simulink subsystem "iLBCTransmit"  (R2024b)
settings: Solver=VariableStepAuto  StartTime=0.0  StopTime=10.0  RelTol=1e-3
values from neighbouring files (symbols this model uses):
  in = pn()    [waveform_generator_Preamble.m]
  LSF = hexToArray(LSF,1)    [Full_transmit.m]
undefined symbols (not defined in the file or in its folder): dspblkCoreblockFVToolHelper, gcbh, ilbc, ilbcMode
libraries: simulink x19, matrix_library x13, dspmtrx3 x9, dspquant2 x6, dspilbclib x5, dspstat3 x5, dspsigops x5, simulink_need_slupdate x2, audiosources x1, dsplp x1, dspsolvers x1
(part 2 of 2)

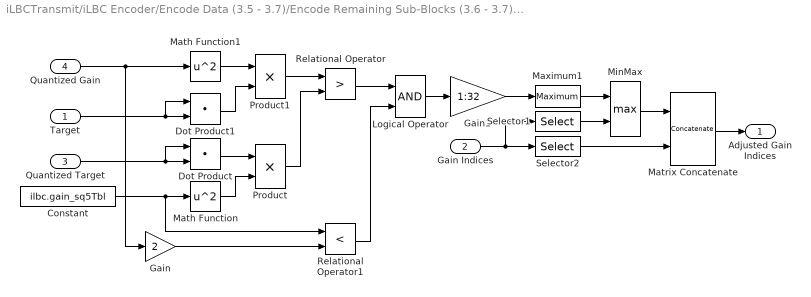
== system iLBCTransmit/iLBC Encoder/Encode Data (3.5 - 3.7)/Encode Remaining Sub-Blocks (3.6 - 3.7)/Encode Sub-Block (3.6.2 - 3.7)/Adjust First Gain Index (3.7) ==
  Target : Inport
  Gain Indices : Inport  Port=2
  Quantized Target : Inport  Port=3
  Quantized Gain : Inport  Port=4
  Constant : Constant  Value=ilbc.gain_sq5Tbl  VectorParams1D=off  OutDataTypeStr=Inherit: Inherit via back propagation
  Dot Product : DotProduct  OutDataTypeStr=Inherit: Inherit via internal rule
  Dot Product1 : DotProduct  OutDataTypeStr=Inherit: Inherit via internal rule
  Gain : Gain  Gain=2
  Gain1 : Gain  Gain=1:32  OutDataTypeStr=Inherit: Inherit via back propagation
  Logical Operator : Logic  AllPortsSameDT=off  OutDataTypeStr=uint(8)
  Math Function : Math  Operator=square  SignedPower=on
  Math Function1 : Math  Operator=square  SignedPower=on
  Matrix Concatenate : Concatenate  Mode=Multidimensional array
  Maximum1 : dspstat3/Maximum  operation=maximum  fcn=Index  indexBase=Zero  operateOver=Each row  Dimension=1  InputProcessing=Columns as channels (frame based)  reset=None  roiEnable=off  roiType=Rectangles  roiPortion=Entire ROI  roiOutput=Individual statistics for each ROI  roiFlag=off  roundingMode=Floor  overflowMode=off  accumDataTypeStr=Inherit: Same as product output  accumLastDataTypeStr=Inherit: Same as product output
  MinMax : MinMax  Function=max  Inputs=2  OutDataTypeStr=Inherit: Inherit via back propagation
  Product : Product  RndMeth=Zero
  Product1 : Product  RndMeth=Zero
  Relational Operator : RelationalOperator  Operator=>  OutDataTypeStr=uint(8)  InputSameDT=off
  Relational Operator1 : RelationalOperator  Operator=<  OutDataTypeStr=uint(8)  InputSameDT=off
  Selector1 : Selector  NumberOfDimensions=2  InputPortWidth=151  IndexOptions=Index vector (dialog),Select all  Indices=1,1  OutputSizes=1,1
  Selector2 : Selector  NumberOfDimensions=2  InputPortWidth=151  IndexOptions=Index vector (dialog),Select all  Indices=2:3,1  OutputSizes=1,1
  Adjusted Gain Indices : Outport  VectorParamsAs1DForOutWhenUnconnected=off
  wires:
  Gain1/1 -> Maximum1/1
  Logical Operator/1 -> Gain1/1
  Relational Operator1/1 -> Logical Operator/2
  Relational Operator/1 -> Logical Operator/1
  Gain/1 -> Relational Operator1/2
  Product/1 -> Relational Operator/2
  Product1/1 -> Relational Operator/1
  Target/1 -> Dot Product1/1, Dot Product1/2
  Quantized Target/1 -> Dot Product/1, Dot Product/2
  Quantized Gain/1 -> Gain/1, Math Function1/1
  Dot Product1/1 -> Product1/2
  Math Function1/1 -> Product1/1
  Dot Product/1 -> Product/1
  Math Function/1 -> Product/2
  Constant/1 -> Relational Operator1/1, Math Function/1
  Matrix Concatenate/1 -> Adjusted Gain Indices/1
  MinMax/1 -> Matrix Concatenate/1
  Maximum1/1 -> MinMax/1
  Selector1/1 -> MinMax/2
  Selector2/1 -> Matrix Concatenate/2
  Gain Indices/1 -> Selector2/1, Selector1/1

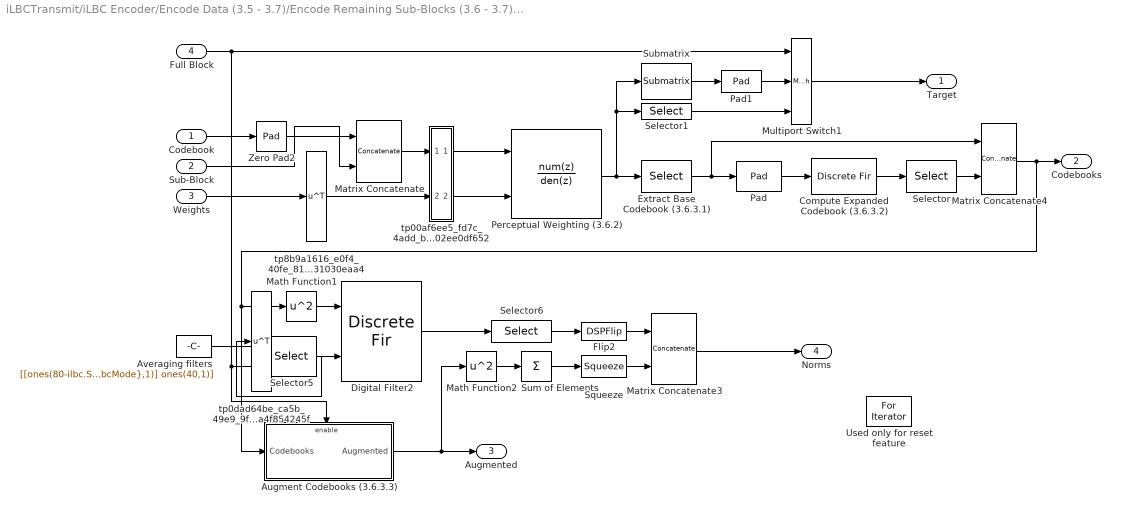
== system iLBCTransmit/iLBC Encoder/Encode Data (3.5 - 3.7)/Encode Remaining Sub-Blocks (3.6 - 3.7)/Encode Sub-Block (3.6.2 - 3.7)/Compute Codebooks (3.6.2 - 3.6.3) ==
  Codebook : Inport
  Sub-Block : Inport  Port=2
  Weights : Inport  Port=3
  Full Block : Inport  Port=4
  Augment Codebooks (3.6.3.3) : Subsystem
  Averaging filters : Constant  Value=[[ones(80-ilbc.STATE_SHORT_LEN{ilbcMode},1); zeros(40-80+ilbc.STATE_SHORT_LEN{ilbcMode},1)] ones(40,1)]  OutDataTypeStr=Inherit: Inherit via back propagation
  Compute Expanded Codebook (3.6.3.2) : DiscreteFir  Coefficients=ilbc.cbfiltersTbl  InputProcessing=Columns as channels (frame based)  AccumDataTypeStr=Inherit: Same as product output
  Digital Filter2 : DiscreteFir  CoefSource=Input port  Coefficients=[1 2]  InputProcessing=Columns as channels (frame based)  AccumDataTypeStr=Inherit: Same as product output
      settings: InputPortMap=u0,u1
  Extract Base Codebook (3.6.3.1) : Selector  NumberOfDimensions=2  InputPortWidth=151  IndexOptions=Index vector (dialog),Index vector (dialog)  Indices=1:147,1  OutputSizes=1,1
  Flip2 : DSPFlip
  Math Function1 : Math  Operator=square  SignedPower=on
  Math Function2 : Math  Operator=square  SignedPower=on
  Matrix Concatenate : Concatenate  Mode=Multidimensional array
  Matrix Concatenate3 : Concatenate  Mode=Multidimensional array
  Matrix Concatenate4 : Concatenate  Mode=Multidimensional array  ConcatenateDimension=2
  Multiport Switch1 : MultiPortSwitch  DataPortOrder=Zero-based contiguous  Inputs=2  zeroidx=on  SaturateOnIntegerOverflow=off  InputSameDT=off
  Pad : dspsigops/Pad  padAlong=Specified dimensions  dimsToPad=1  valSrc=Specify via dialog  padVal=0  spec=Pad size  padNumOutRowsSpecMethod=User-specified  numOutRows=1  padNumOutColsSpecMethod=User-specified  numOutCols=1  isVarDimsMode=off  padBeginning=0  padEnd=4  outSizeMode=User-specified  outSize=1  padSigAt=End  trunc_flag=None  roundingMode=Floor  overflowMode=off  truncOrWrapMode=Truncate  wrap_flag=None
  Pad1 : dspsigops/Pad  padAlong=Columns  dimsToPad=1  valSrc=Specify via dialog  padVal=0  spec=Output size  padNumOutRowsSpecMethod=User-specified  numOutRows=40  padNumOutColsSpecMethod=User-specified  numOutCols=1  isVarDimsMode=off  padBeginning=0  padEnd=0  outSizeMode=User-specified  outSize=1  padSigAt=Beginning  trunc_flag=None  roundingMode=Floor  overflowMode=off  truncOrWrapMode=Truncate  wrap_flag=None
  Perceptual Weighting (3.6.2) : DiscreteFilter  Numerator=1  DenominatorSource=Input port  Denominator=[1 0.1]  InputProcessing=Columns as channels (frame based)  a0EqualsOne=on
      settings: InputPortMap=u0,p3
  Selector : Selector  NumberOfDimensions=2  InputPortWidth=151  IndexOptions=Index vector (dialog),Index vector (dialog)  Indices=5:151,1  OutputSizes=1,1
  Selector1 : Selector  NumberOfDimensions=2  InputPortWidth=151  IndexOptions=Index vector (dialog),Index vector (dialog)  Indices=148:187,1  OutputSizes=1,1
  Selector5 : Selector  NumberOfDimensions=2  IndexMode=Zero-based  InputPortWidth=3  IndexOptions=Select all,Index vector (port)  Indices=[1 3],1  OutputSizes=1,1
  Selector6 : Selector  NumberOfDimensions=2  InputPortWidth=3  IndexOptions=Index vector (dialog),Select all  Indices=40:147,1  OutputSizes=1,1
  Squeeze : Squeeze
  Submatrix : matrix_library/Submatrix  RowSpan=Range of rows  RowStartMode=Index  RowStartIndex=148  RowEndMode=Index  RowEndIndex=147+(80-ilbc.STATE_SHORT_LEN{ilbcMode})  ColSpan=All columns  ColStartMode=First  ColStartIndex=1  ColEndMode=Last  ColEndIndex=1
  Sum of Elements : Sum  Inputs=+  CollapseMode=Specified dimension  CollapseDim=2
  Used only for reset feature : ForIterator  ResetStates=reset  IterationLimit=1  ShowIterationPort=off
  Zero Pad2 : dspsigops/Pad  padAlong=Columns  dimsToPad=1  valSrc=Specify via dialog  padVal=0  spec=Output size  padNumOutRowsSpecMethod=User-specified  numOutRows=147  padNumOutColsSpecMethod=User-specified  numOutCols=1  isVarDimsMode=off  padBeginning=0  padEnd=0  outSizeMode=User-specified  outSize=1  padSigAt=Beginning  trunc_flag=None  roundingMode=Floor  overflowMode=off  truncOrWrapMode=Truncate  wrap_flag=None
  tp00af6ee5_fd7c_4add_bbb5_3302ee0df652 : Subsystem
  tp0dad64be_ca5b_49e9_9fd5_44a4f854245f : Math  Operator=transpose  SignedPower=on
  tp8b9a1616_e0f4_40fe_814a_bea31030eaa4 : Math  Operator=transpose  SignedPower=on
  Target : Outport  VectorParamsAs1DForOutWhenUnconnected=off
  Codebooks : Outport  Port=2  VectorParamsAs1DForOutWhenUnconnected=off
  Augmented : Outport  Port=3  VectorParamsAs1DForOutWhenUnconnected=off
  Norms : Outport  Port=4  VectorParamsAs1DForOutWhenUnconnected=off
  wires:
  Matrix Concatenate3/1 -> Norms/1
  tp00af6ee5_fd7c_4add_bbb5_3302ee0df652/2(scaled den) -> Perceptual Weighting (3.6.2)/2
  tp8b9a1616_e0f4_40fe_814a_bea31030eaa4/1 -> tp00af6ee5_fd7c_4add_bbb5_3302ee0df652/2(den)
  tp00af6ee5_fd7c_4add_bbb5_3302ee0df652/1(scaled in) -> Perceptual Weighting (3.6.2)/1
  Matrix Concatenate/1 -> tp00af6ee5_fd7c_4add_bbb5_3302ee0df652/1(in)
  Weights/1 -> tp8b9a1616_e0f4_40fe_814a_bea31030eaa4/1
  tp0dad64be_ca5b_49e9_9fd5_44a4f854245f/1 -> Digital Filter2/2
  Selector5/1 -> tp0dad64be_ca5b_49e9_9fd5_44a4f854245f/1
  Selector1/1 -> Multiport Switch1/3
  Pad1/1 -> Multiport Switch1/2
  Flip2/1 -> Matrix Concatenate3/1
  Pad/1 -> Compute Expanded Codebook (3.6.3.2)/1
  Zero Pad2/1 -> Matrix Concatenate/1
  Sub-Block/1 -> Matrix Concatenate/2
  Codebook/1 -> Zero Pad2/1
  Averaging filters/1 -> Selector5/1
  Selector6/1 -> Flip2/1
  Digital Filter2/1 -> Selector6/1
  Math Function1/1 -> Digital Filter2/1
  Extract Base Codebook (3.6.3.1)/1 -> Matrix Concatenate4/1, Pad/1
  Perceptual Weighting (3.6.2)/1 -> Extract Base Codebook (3.6.3.1)/1, Submatrix/1, Selector1/1
  Full Block/1 -> Multiport Switch1/1, Selector5/2, Augment Codebooks (3.6.3.3)/Enable
  Multiport Switch1/1 -> Target/1
  Math Function2/1 -> Sum of Elements/1
  Sum of Elements/1 -> Squeeze/1
  Submatrix/1 -> Pad1/1
  Compute Expanded Codebook (3.6.3.2)/1 -> Selector/1
  Matrix Concatenate4/1 -> Codebooks/1, Augment Codebooks (3.6.3.3)/1(Codebooks), Math Function1/1
  Augment Codebooks (3.6.3.3)/1(Augmented) -> Math Function2/1, Augmented/1
  Squeeze/1 -> Matrix Concatenate3/2
  Selector/1 -> Matrix Concatenate4/2

== system iLBCTransmit/iLBC Encoder/Encode Data (3.5 - 3.7)/Extract Sub-Blocks (3.5.1) and Sort LPC Filters/Parse Blocks/Flip Full Blocks ==
  Sub-blocks : Inport
  Start State Number : Inport  Port=2
  Assignment : Assignment  NumberOfDimensions=2  IndexMode=Zero-based  OutputInitialize=Specify size for each dimension in table  IndexOptions=Assign all,Index vector (port)  Indices=-1,1  OutputSizes=40,ilbc.NSUB{ilbcMode}-2
  Constant : Constant  Value=ilbc.NSUB{ilbcMode}-2  OutDataTypeStr=Inherit: Inherit via back propagation
  Flip1 : DSPFlip
  For Iterator : ForIterator  IterationLimit=ilbc.NSUB{ilbcMode}-2  IndexMode=Zero-based
  Multiport Switch2 : MultiPortSwitch  DataPortOrder=Zero-based contiguous  Inputs=2  zeroidx=on  SaturateOnIntegerOverflow=off  InputSameDT=off
  Relational Operator : RelationalOperator  OutDataTypeStr=boolean  InputSameDT=off
  Selector1 : Selector  NumberOfDimensions=2  IndexMode=Zero-based  InputPortWidth=3  IndexOptions=Select all,Index vector (port)  Indices=-1,-1  OutputSizes=1
  Sum : Sum  Inputs=+-|
  Flipped : Outport  VectorParamsAs1DForOutWhenUnconnected=off
  wires:
  Sub-blocks/1 -> Selector1/1
  Selector1/1 -> Flip1/1, Multiport Switch2/3
  Multiport Switch2/1 -> Assignment/1
  Assignment/1 -> Flipped/1
  Flip1/1 -> Multiport Switch2/2
  Relational Operator/1 -> Multiport Switch2/1
  Sum/1 -> Relational Operator/1
  Start State Number/1 -> Relational Operator/2
  Constant/1 -> Sum/1
  For Iterator/1 -> Sum/2, Selector1/2, Assignment/2

== system iLBCTransmit/iLBC Encoder/Encode Data (3.5 - 3.7)/Encode Remaining Sub-Blocks (3.6 - 3.7)/Encode Sub-Block (3.6.2 - 3.7)/3 Stage Sub-Block Encoder (3.6.4)/Compute Correlations (3.6.4.1) ==
  Codebooks : Inport
  Augmented : Inport  Port=2
  Target : Inport  Port=3
  Array-Vector Multiply : dspmtrx3/Array-Vector Multiply  mode=Mute  saveAsFlag=0  Dimension=2  V_Source=Input port  V_VectFromMask=[0.5 0.25]  roundingMode=Floor  overflowMode=off  firstCoeffSignedness=Auto  firstCoeffDataTypeStr=Inherit: Same word length as input  firstCoeffMin=[]  firstCoeffMax=[]  firstCoeffLastDataTypeStr=Inherit: Same word length as input  prodOutputSignedness=Auto  accumSignedness=Auto  outputSignedness=Auto  outputDataTypeStr=Inherit: Same as product output  outputMin=[]  outputMax=[]  outputLastDataTypeStr=Inherit: Same as product output
  Digital Filter : DiscreteFir  CoefSource=Input port  Coefficients=[1 2]  InputProcessing=Columns as channels (frame based)  AccumDataTypeStr=Inherit: Same as product output
      settings: InputPortMap=u0,u1
  Flip : DSPFlip
  Flip1 : DSPFlip
  Matrix Concatenate1 : Concatenate  Mode=Multidimensional array
  Squeeze : Squeeze
  Submatrix : matrix_library/Submatrix  RowSpan=Range of rows  RowStartMode=Offset from last  RowStartIndex=107  RowEndMode=Last  RowEndIndex=1  ColSpan=All columns  ColStartMode=First  ColStartIndex=1  ColEndMode=Last  ColEndIndex=1
  Sum of Elements : Sum  Inputs=+  CollapseMode=Specified dimension  CollapseDim=2
  tp6aab9b3f_7577_43e6_a5f1_9324e7fa3d31 : Math  Operator=transpose  SignedPower=on
  Correlations : Outport  VectorParamsAs1DForOutWhenUnconnected=off
  wires:
  tp6aab9b3f_7577_43e6_a5f1_9324e7fa3d31/1 -> Digital Filter/2
  Flip/1 -> tp6aab9b3f_7577_43e6_a5f1_9324e7fa3d31/1
  Target/1 -> Flip/1, Array-Vector Multiply/2
  Sum of Elements/1 -> Squeeze/1
  Codebooks/1 -> Digital Filter/1
  Augmented/1 -> Array-Vector Multiply/1
  Digital Filter/1 -> Submatrix/1
  Flip1/1 -> Matrix Concatenate1/1
  Submatrix/1 -> Flip1/1
  Matrix Concatenate1/1 -> Correlations/1
  Array-Vector Multiply/1 -> Sum of Elements/1
  Squeeze/1 -> Matrix Concatenate1/2

== system iLBCTransmit/iLBC Encoder/Encode Data (3.5 - 3.7)/Encode Remaining Sub-Blocks (3.6 - 3.7)/Encode Sub-Block (3.6.2 - 3.7)/3 Stage Sub-Block Encoder (3.6.4)/Encode Gain (3.6.4.2) ==
  Stage : Inport
  Gain Value : Inport  Port=2
  Last Quantized Gain : Inport  Port=3
  Abs : Abs  OutDataTypeStr=Inherit: Inherit via back propagation  SaturateOnIntegerOverflow=off
  Constant1 : Constant  Value=[ilbc.gain_sq5Tbl; ilbc.gain_sq4Tbl; ilbc.gain_sq3Tbl]  VectorParams1D=off  OutDataTypeStr=Inherit: Inherit via back propagation
  Data Type Duplicate1 : DataTypeDuplicate
  Product : Product  OutDataTypeStr=Inherit: Inherit via back propagation  RndMeth=Zero
  Saturation1 : Saturate  UpperLimit=inf  LowerLimit=0.1  OutDataTypeStr=Inherit: Inherit via back propagation
  Selector1 : Selector  NumberOfDimensions=2  IndexMode=Zero-based  InputPortWidth=3  IndexOptions=Index vector (port),Select all  Indices=1,1  OutputSizes=1,1
  VQ Encoder : dspquant2/Vector Quantizer Encoder  CBsource=Input port  codebook=GainCBs{Iteration}  distMeasure=Squared error  wgtSrc=Specify via dialog  weights=[1 1 1]  tieBreakRule=Choose the lower index  outQU=on  outQError=off  idtype=uint8  roundingMode=Floor  overflowMode=off
  Gain Index : Outport  VectorParamsAs1DForOutWhenUnconnected=off
  Quantized Gain : Outport  Port=2  VectorParamsAs1DForOutWhenUnconnected=off
  wires:
  Last Quantized Gain/1 -> Abs/1, Data Type Duplicate1/1
  Saturation1/1 -> Product/2
  Abs/1 -> Saturation1/1
  Product/1 -> VQ Encoder/2
  VQ Encoder/1 -> Gain Index/1
  VQ Encoder/2 -> Quantized Gain/1
  Gain Value/1 -> VQ Encoder/1
  Selector1/1 -> Product/1
  Constant1/1 -> Selector1/1, Data Type Duplicate1/2
  Stage/1 -> Selector1/2

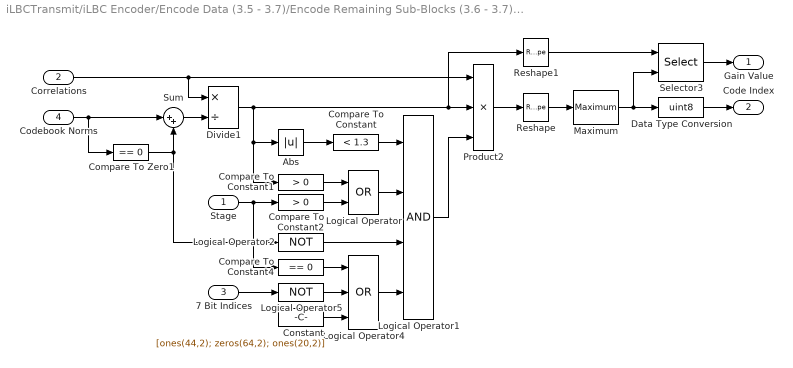
== system iLBCTransmit/iLBC Encoder/Encode Data (3.5 - 3.7)/Encode Remaining Sub-Blocks (3.6 - 3.7)/Encode Sub-Block (3.6.2 - 3.7)/3 Stage Sub-Block Encoder (3.6.4)/Search Codebooks (3.6.4.1 continued) ==
  Stage : Inport
  Correlations : Inport  Port=2
  7 Bit Indices : Inport  Port=3
  Codebook Norms : Inport  Port=4
  Abs : Abs  SaturateOnIntegerOverflow=off
  Compare To Constant : simulink/Logic and Bit Operations/Compare To Constant  relop=<  const=1.3  OutDataTypeStr=boolean  ZeroCross=off
  Compare To Constant1 : simulink/Logic and Bit Operations/Compare To Constant  relop=>  const=0  OutDataTypeStr=boolean  ZeroCross=off
  Compare To Constant2 : simulink/Logic and Bit Operations/Compare To Constant  relop=>  const=0  OutDataTypeStr=boolean  ZeroCross=off
  Compare To Constant4 : simulink/Logic and Bit Operations/Compare To Constant  relop===  const=0  OutDataTypeStr=boolean  ZeroCross=off
  Compare To Zero1 : simulink/Logic and Bit Operations/Compare To Zero  relop===  OutDataTypeStr=boolean  ZeroCross=off
  Constant : Constant  Value=[ones(44,2); zeros(64,2); ones(20,2)]  VectorParams1D=off  OutDataTypeStr=Inherit: Inherit via back propagation
  Data Type Conversion : DataTypeConversion  OutDataTypeStr=uint8  SaturateOnIntegerOverflow=off  RndMeth=Floor
  Divide1 : Product  Inputs=*/  OutDataTypeStr=Inherit: Same as first input
  Logical Operator : Logic  Operator=OR  AllPortsSameDT=off  OutDataTypeStr=boolean
  Logical Operator1 : Logic  Inputs=4  AllPortsSameDT=off  OutDataTypeStr=boolean
  Logical Operator2 : Logic  Operator=NOT  AllPortsSameDT=off  OutDataTypeStr=boolean
  Logical Operator4 : Logic  Operator=OR  Inputs=3  AllPortsSameDT=off  OutDataTypeStr=boolean
  Logical Operator5 : Logic  Operator=NOT  AllPortsSameDT=off  OutDataTypeStr=boolean
  Maximum : dspstat3/Maximum  operation=maximum  fcn=Index  indexBase=Zero  operateOver=Each column  Dimension=1  InputProcessing=Columns as channels (frame based)  reset=None  roiEnable=off  roiType=Rectangles  roiPortion=Entire ROI  roiOutput=Individual statistics for each ROI  roiFlag=off  roundingMode=Floor  overflowMode=off  accumDataTypeStr=Inherit: Same as product output  accumLastDataTypeStr=Inherit: Same as product output
  Product2 : Product  Inputs=3  RndMeth=Zero  OutDataTypeStr=Inherit: Same as first input
  Reshape : Reshape  OutputDimensionality=Column vector (2-D)
  Reshape1 : Reshape  OutputDimensionality=Column vector (2-D)
  Selector3 : Selector  NumberOfDimensions=2  IndexMode=Zero-based  InputPortWidth=3  IndexOptions=Index vector (port),Select all  Indices=1,1  OutputSizes=1,1
  Sum : Sum  Inputs=|++  OutDataTypeStr=Inherit: Same as first input
  Gain Value : Outport  VectorParamsAs1DForOutWhenUnconnected=off
  Code Index : Outport  Port=2  VectorParamsAs1DForOutWhenUnconnected=off
  wires:
  Abs/1 -> Compare To Constant/1
  Codebook Norms/1 -> Compare To Zero1/1, Sum/1
  Data Type Conversion/1 -> Code Index/1
  Product2/1 -> Reshape/1
  Selector3/1 -> Gain Value/1
  Sum/1 -> Divide1/2
  Compare To Zero1/1 -> Sum/2, Logical Operator2/1
  Maximum/1 -> Data Type Conversion/1, Selector3/2
  Correlations/1 -> Divide1/1, Product2/1
  Compare To Constant/1 -> Logical Operator1/1
  Logical Operator4/1 -> Logical Operator1/4
  7 Bit Indices/1 -> Logical Operator5/1
  Stage/1 -> Compare To Constant2/1, Compare To Constant4/1
  Reshape/1 -> Maximum/1
  Reshape1/1 -> Selector3/1
  Compare To Constant4/1 -> Logical Operator4/1
  Logical Operator5/1 -> Logical Operator4/2
  Constant/1 -> Logical Operator4/3
  Compare To Constant1/1 -> Logical Operator/1
  Compare To Constant2/1 -> Logical Operator/2
  Logical Operator/1 -> Logical Operator1/2
  Logical Operator2/1 -> Logical Operator1/3
  Logical Operator1/1 -> Product2/3
  Divide1/1 -> Product2/2, Reshape1/1, Abs/1, Compare To Constant1/1

== system iLBCTransmit/iLBC Encoder/Encode Data (3.5 - 3.7)/Encode Remaining Sub-Blocks (3.6 - 3.7)/Encode Sub-Block (3.6.2 - 3.7)/Compute Codebooks (3.6.2 - 3.6.3)/Augment Codebooks (3.6.3.3) ==
  Codebooks : Inport
  Enable : EnablePort
  Compute Augmented CB : Subsystem  TreatAsAtomicUnit=on
  Matrix Scaling1 : dspmtrx3/Array-Vector Multiply  mode=Mute  saveAsFlag=0  Dimension=1  V_Source=Dialog parameter  V_VectFromMask=[1 0.8 0.6 0.4 0.2]  roundingMode=Floor  overflowMode=off  firstCoeffSignedness=Auto  firstCoeffDataTypeStr=Inherit: Same word length as input  firstCoeffMin=[]  firstCoeffMax=[]  firstCoeffLastDataTypeStr=Inherit: Same word length as input  prodOutputSignedness=Auto  accumSignedness=Auto  outputSignedness=Auto  outputDataTypeStr=Inherit: Same as product output  outputMin=[]  outputMax=[]  outputLastDataTypeStr=Inherit: Same as product output
  Selector3 : Selector  NumberOfDimensions=2  InputPortWidth=3  IndexOptions=Index vector (dialog),Select all  Indices=[143:147],1  OutputSizes=1,1
  Augmented : Outport  OutputWhenDisabled=reset  InitialOutput=zeros(20,40,2)  VectorParamsAs1DForOutWhenUnconnected=off
  wires:
  Selector3/1 -> Matrix Scaling1/1
  Matrix Scaling1/1 -> Compute Augmented CB/2(Interpolation)
  Codebooks/1 -> Selector3/1, Compute Augmented CB/1(Codebook)
  Compute Augmented CB/1(Augmented) -> Augmented/1

== system iLBCTransmit/iLBC Encoder/Encode Data (3.5 - 3.7)/Encode Remaining Sub-Blocks (3.6 - 3.7)/Encode Sub-Block (3.6.2 - 3.7)/Compute Codebooks (3.6.2 - 3.6.3)/tp00af6ee5_fd7c_4add_bbb5_3302ee0df652 ==
  in : Inport
  den : Inport  Port=2
  Scale Denominator : Product  Inputs=*/
  Scale in : Product  Inputs=*/
  Select a0 : matrix_library/Submatrix  RowSpan=Range of rows  RowStartMode=First  RowStartIndex=1  RowEndMode=Index  RowEndIndex=1  ColSpan=Range of columns  ColStartMode=First  ColStartIndex=1  ColEndMode=Index  ColEndIndex=1
  scaled in : Outport  VectorParamsAs1DForOutWhenUnconnected=off
  scaled den : Outport  Port=2  VectorParamsAs1DForOutWhenUnconnected=off
  wires:
  Scale Denominator/1 -> scaled den/1
  Scale in/1 -> scaled in/1
  Select a0/1 -> Scale Denominator/2, Scale in/2
  in/1 -> Scale in/1
  den/1 -> Scale Denominator/1, Select a0/1

== system iLBCTransmit/iLBC Encoder/Encode Data (3.5 - 3.7)/Encode Remaining Sub-Blocks (3.6 - 3.7)/Encode Sub-Block (3.6.2 - 3.7)/Compute Codebooks (3.6.2 - 3.6.3)/Augment Codebooks (3.6.3.3)/Compute Augmented CB ==
  Codebook : Inport
  Interpolation : Inport  Port=2
  Assignment1 : Assignment  NumberOfDimensions=3  OutputInitialize=Specify size for each dimension in table  IndexOptions=Index vector (port),Assign all,Assign all  Indices=1,1,1  OutputSizes=20,40,2
  Bias : Bias  Bias=15  SaturateOnIntegerOverflow=off
  Compute Code : Subsystem
  Constant : Constant  Value=ilbc.augmented_idxTbl  VectorParams1D=off  OutDataTypeStr=uint8
  For Iterator : ForIterator  IterationLimit=20  IterationVariableDataType=int8
  Matrix Scaling : dspmtrx3/Array-Vector Multiply  mode=Mute  saveAsFlag=0  Dimension=1  V_Source=Dialog parameter  V_VectFromMask=[0 0.2 0.4 0.6 0.8]  roundingMode=Floor  overflowMode=off  firstCoeffSignedness=Auto  firstCoeffDataTypeStr=Inherit: Same word length as input  firstCoeffMin=[]  firstCoeffMax=[]  firstCoeffLastDataTypeStr=Inherit: Same word length as input  prodOutputSignedness=Auto  accumSignedness=Auto  outputSignedness=Auto  outputDataTypeStr=Inherit: Same as product output  outputMin=[]  outputMax=[]  outputLastDataTypeStr=Inherit: Same as product output
  Reshape : Reshape  OutputDimensionality=Customize  OutputDimensions=[1 40 2]
  Selector1 : Selector  NumberOfDimensions=2  InputPortWidth=3  IndexOptions=Index vector (port),Select all  Indices=[1 3],1  OutputSizes=1,1
  Selector2 : Selector  NumberOfDimensions=2  InputPortWidth=3  IndexOptions=Starting index (port),Select all  Indices=[1 3],1  OutputSizes=5,1
  Selector3 : Selector  NumberOfDimensions=2  InputPortWidth=3  IndexOptions=Select all,Index vector (port)  Indices=[1 3],1  OutputSizes=1,1
  Sum : Sum  Inputs=++|
  Augmented : Outport  VectorParamsAs1DForOutWhenUnconnected=off
  wires:
  Sum/1 -> Compute Code/2(U)
  Compute Code/1(Y) -> Reshape/1
  For Iterator/1 -> Bias/1, Assignment1/2, Selector3/2
  Codebook/1 -> Selector1/1
  Selector2/1 -> Matrix Scaling/1
  Bias/1 -> Selector2/2, Compute Code/3(Idx1)
  Selector1/1 -> Selector2/1, Compute Code/1(Y0)
  Selector3/1 -> Selector1/2
  Matrix Scaling/1 -> Sum/2
  Interpolation/1 -> Sum/1
  Assignment1/1 -> Augmented/1
  Reshape/1 -> Assignment1/1
  Constant/1 -> Selector3/1

== system iLBCTransmit/iLBC Encoder/Encode Data (3.5 - 3.7)/Encode Remaining Sub-Blocks (3.6 - 3.7)/Encode Sub-Block (3.6.2 - 3.7)/Compute Codebooks (3.6.2 - 3.6.3)/Augment Codebooks (3.6.3.3)/Compute Augmented CB/Compute Code ==
  Y0 : Inport
  U : Inport  Port=2
  Idx1 : Inport  Port=3
  Assignment : Assignment  NumberOfDimensions=2  IndexOptions=Starting index (port),Assign all  Indices=1,1  OutputSizes=40,1
  Used for reset feature only : ForIterator  ResetStates=reset  IterationLimit=1  ShowIterationPort=off  IterationVariableDataType=int8
  Y : Outport  VectorParamsAs1DForOutWhenUnconnected=off
  wires:
  Y0/1 -> Assignment/1
  Idx1/1 -> Assignment/3
  U/1 -> Assignment/2
  Assignment/1 -> Y/1
